simulink model "HumRob_V8"  (R2018a)
settings: Solver=FixedStepDiscrete  StartTime=0.0  StopTime=30  FixedStep=SampleTime  RelTol=1e-3  EnableMultiTasking=on
model workspace (MAT data in the model file):
  sampleTime = Simulink.Parameter
  sampleTime.DataType = 'auto'
  sampleTime.Dimensions = [0 0]
values from neighbouring files (symbols this model uses):
  PHI_t = deg2rad(15)    [init.m]
  scaling = 100    [init.m]
  T_la = 0.2*scaling    (= 20)    [init.m]
  T_st = 0.4*scaling    (= 40)    [init.m]
  T_sw = 1.1*scaling    (= 110)    [init.m]
  T_ta = 0.3*scaling    (= 30)    [init.m]
undefined symbols (not defined in the file or in its folder): DiscIntNeverNeededParam
libraries: raspberrypilib x3, embdlinuxlib x2, simulink x1, dspswit3 x1
settings Model: SimulationMode=external  ExtModeEnableFloating=off  Creator=t21st  LastModifiedBy=Kevin
settings SolverCC: PositivePriorityOrder=on  AutoInsertRateTranBlk=on  InsertRTBMode=Never (minimum delay)
settings DataIOCC: LimitDataPoints=on  MaxDataPoints=1000000
settings OptimizationCC: EnhancedBackFolding=on  PassReuseOutputArgsAs=Individual arguments  MaxStackSize=64  OptimizeBlockOrder=speed  DifferentSizesBufferReuse=on  OptimizationCustomize=off
settings DebuggingCC: ParameterTunabilityLossMsg=error
settings HardwareCC: ProdBitPerPointer=32  ProdBitPerSizeT=32  ProdBitPerPtrDiffT=32  ProdLargestAtomicInteger=Long  ProdLargestAtomicFloat=Double  ProdWordSize=32  ProdHWDeviceType=ARM Compatible->ARM Cortex
settings SFSimCC: MATLABDynamicMemAlloc=off
settings RTWCC: SystemTargetFile=ert.tlc  HardwareBoard=Raspberry Pi  TLCOptions="-aInlineSetEventsForThisBaseRateFcn=TLC_FALSE -aSuppressMultiTaskScheduler=TLC_FALSE  -aRateBasedStepFcn=0"  TemplateMakefile=ert_default_tmf  GenerateReport=on  Toolchain=GNU GCC Raspberry Pi  BuildConfiguration=Faster Runs  IncludeHyperlinkInReport=on  LaunchReport=on  GenerateTraceInfo=on  GenerateTraceReport=on  GenerateTraceReportSl=on  GenerateTraceReportSf=on  GenerateTraceReportEml=on
settings CodeAppCC: ForceParamTrailComments=on  IgnoreCustomStorageClasses=off  OperatorAnnotations=on  SimulinkDataObjDesc=on  SFDataObjDesc=on  InsertBlockDesc=on
settings ERTTargetCC: MatFileLogging=on  SupportVariableSizeSignals=on

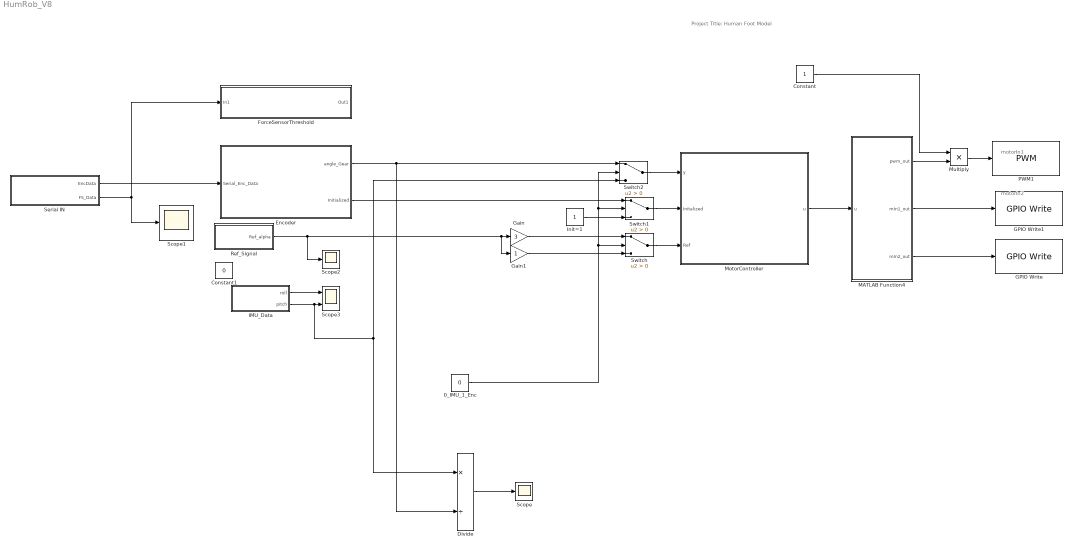
== system HumRob_V8 ==
  note: motorIn1
  note: motorIn2
  note: Project Title: Human Foot Model
  0_IMU_1_Enc : Constant  Value=0
  Constant : Constant
  Constant1 : Constant  Value=0
  Divide : Product  Inputs=*/
  Encoder : Subsystem
  ForceSensorThreshold : Subsystem
  GPIO Write : embdlinuxlib/GPIO Write  Description=asdf  board=Pi 3 Model B  gpio=24  direction=Output  blockPlatform=Raspberry Pi
      settings: SourceProductName=Simulink Support Package for Raspberry Pi Hardware  SourceProductBaseCode=RASPPI
  GPIO Write1 : embdlinuxlib/GPIO Write  board=Pi 3 Model B  gpio=23  direction=Output  blockPlatform=Raspberry Pi
      settings: SourceProductName=Simulink Support Package for Raspberry Pi Hardware  SourceProductBaseCode=RASPPI
  Gain : Gain  Gain=3
  Gain1 : Gain
  IMU_Data : Subsystem
  Init=1 : Constant
  MATLAB Function4 : MATLAB Function  TreatAsAtomicUnit=on
  MotorController : Subsystem
  Multiply : Product
  PWM1 : raspberrypilib/PWM  board=Pi 3 Model B  Pin_=18  Frequency=1000  blockPlatform=Raspberry Pi
      settings: SourceProductName=Simulink Support Package for Raspberry Pi Hardware  SourceProductBaseCode=RASPPI
  Ref_Signal : Subsystem
  Scope : Scope
  Scope1 : Scope
  Scope2 : Scope
  Scope3 : Scope  NumInputPorts=2
  Serial IN : Subsystem
  Switch : Switch  Criteria=u2 > Threshold
  Switch1 : Switch  Criteria=u2 > Threshold
  Switch2 : Switch  Criteria=u2 > Threshold
  wires:
  MATLAB Function4/2(mIn1_out) -> GPIO Write1/1
  MATLAB Function4/3(mIn2_out) -> GPIO Write/1
  MATLAB Function4/1(pwm_out) -> Multiply/2
  Multiply/1 -> PWM1/1
  Encoder/1("angle_Gear ") -> Switch2/1, Divide/2
  Encoder/2(Initialized) -> Switch1/1
  Gain/1 -> Switch/1
  MotorController/1(u) -> MATLAB Function4/1(u)
  Serial IN/2(FS_Data) -> ForceSensorThreshold/1(In1), Scope1/1
  Ref_Signal/1(Ref_alpha) -> Scope2/1, Gain1/1, Gain/1
  Serial IN/1("EncData ") -> Encoder/1(Serial_Enc_Data)
  IMU_Data/2(pitch) -> Divide/1, Switch2/3, Scope3/2
  IMU_Data/1(roll) -> Scope3/1
  Constant/1 -> Multiply/1
  Switch/1 -> MotorController/3(Ref)
  Gain1/1 -> Switch/3
  0_IMU_1_Enc/1 -> Switch2/2, Switch1/2, Switch/2
  Init=1/1 -> Switch1/3
  Switch2/1 -> MotorController/1(y)
  Switch1/1 -> MotorController/2(Initalized)
  Divide/1 -> Scope/1

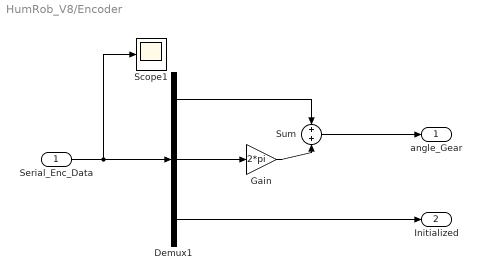
== system HumRob_V8/Encoder ==
  Serial_Enc_Data : Inport
  Demux1 : Demux  Outputs=3
  Gain : Gain  Gain=2*pi
  Scope1 : Scope
  Sum : Sum  Inputs=+|+
  "angle_Gear " : Outport
  Initialized : Outport  Port=2
  wires:
  Demux1/2 -> Gain/1
  Demux1/1 -> Sum/1
  Gain/1 -> Sum/2
  Sum/1 -> "angle_Gear "/1
  Demux1/3 -> Initialized/1
  Serial_Enc_Data/1 -> Scope1/1, Demux1/1

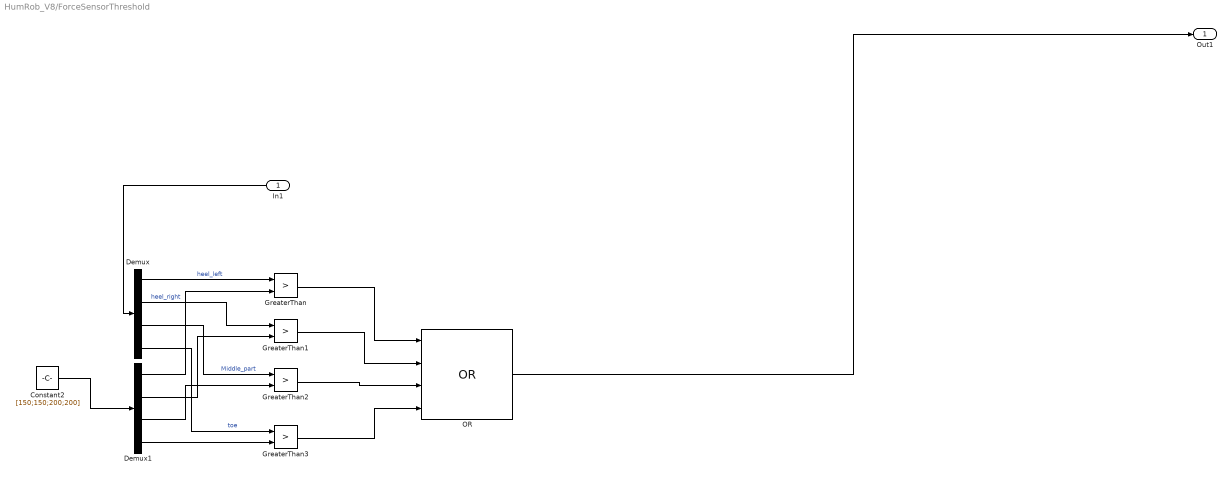
== system HumRob_V8/ForceSensorThreshold ==
  In1 : Inport
  Constant2 : Constant  Value=[150;150;200;200]
  Demux : Demux
  Demux1 : Demux
  GreaterThan{,1..3} (4 alike) : RelationalOperator  Operator=>  OutDataTypeStr=boolean  RndMeth=Simplest
  OR : Logic  Operator=OR  Inputs=4  IconShape=distinctive  AllPortsSameDT=off  OutDataTypeStr=boolean
  Out1 : Outport
  wires:
  Demux/3 -> GreaterThan2/1  "Middle_part"
  Demux1/2 -> GreaterThan1/2
  GreaterThan3/1 -> OR/4
  Demux/4 -> GreaterThan3/1  "toe"
  GreaterThan2/1 -> OR/3
  GreaterThan1/1 -> OR/2
  Demux/2 -> GreaterThan1/1  "heel_right"
  GreaterThan/1 -> OR/1
  Demux1/1 -> GreaterThan/2
  Demux/1 -> GreaterThan/1  "heel_left"
  Demux1/3 -> GreaterThan2/2
  Demux1/4 -> GreaterThan3/2
  OR/1 -> Out1/1
  Constant2/1 -> Demux1/1
  In1/1 -> Demux/1

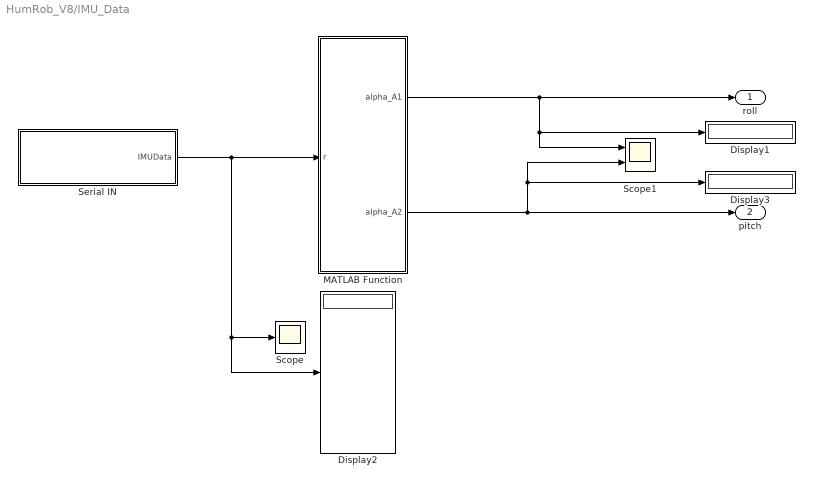
== system HumRob_V8/IMU_Data ==
  Display1 : Display
  Display2 : Display
  Display3 : Display
  MATLAB Function : MATLAB Function  TreatAsAtomicUnit=on
  Scope : Scope
  Scope1 : Scope  NumInputPorts=2
  Serial IN : Subsystem
  roll : Outport
  pitch : Outport  Port=2
  wires:
  Serial IN/1("IMUData ") -> Scope/1, Display2/1, MATLAB Function/1(r)
  MATLAB Function/1(alpha_A1) -> roll/1, Scope1/1, Display1/1
  MATLAB Function/2(alpha_A2) -> pitch/1, Scope1/2, Display3/1

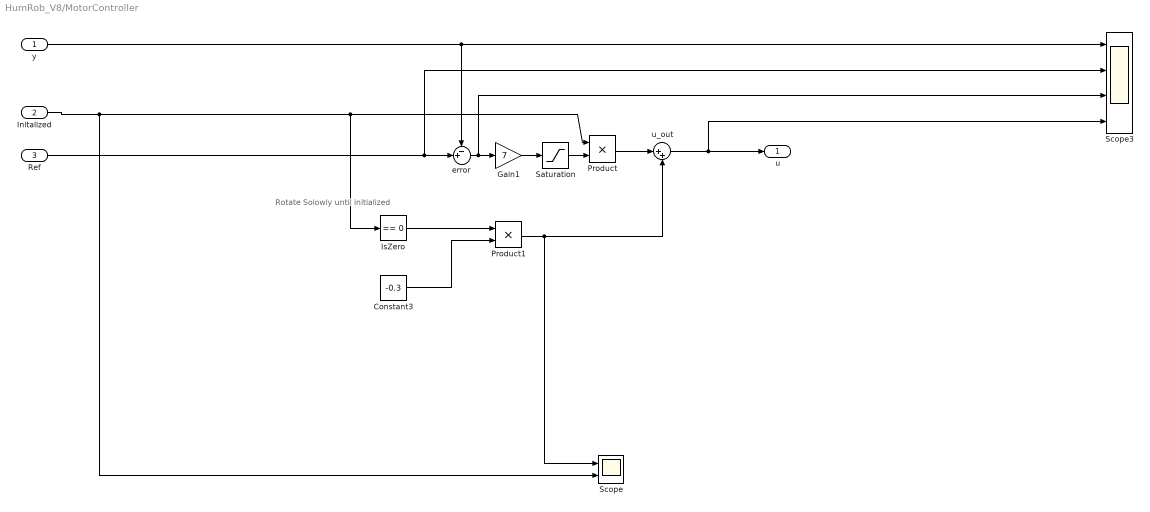
== system HumRob_V8/MotorController ==
  note: Rotate Solowly until initialized
  y : Inport
  Initalized : Inport  Port=2
  Ref : Inport  Port=3
  Constant3 : Constant  Value=-0.3
  Gain1 : Gain  Gain=7
  IsZero : simulink/Logic and Bit Operations/Compare To Zero  relop===  OutDataTypeStr=boolean
  Product : Product
  Product1 : Product
  Saturation : Saturate  UpperLimit=1  LowerLimit=-1
  Scope : Scope  NumInputPorts=2
  Scope3 : Scope  NumInputPorts=4
  error : Sum  Inputs=-+|
  u_out : Sum  Inputs=|++
  u : Outport
  wires:
  Gain1/1 -> Saturation/1
  Product/1 -> u_out/1
  error/1 -> Scope3/3, Gain1/1
  Saturation/1 -> Product/2
  y/1 -> error/1, Scope3/1
  Product1/1 -> Scope/1, u_out/2
  u_out/1 -> Scope3/4, u/1
  Constant3/1 -> Product1/2
  IsZero/1 -> Product1/1
  Ref/1 -> Scope3/2, error/2
  Initalized/1 -> Scope/2, IsZero/1, Product/1

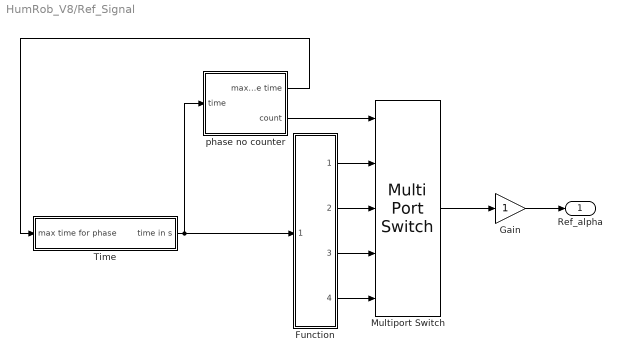
== system HumRob_V8/Ref_Signal ==
  Function : Subsystem
  Gain : Gain
  Multiport Switch : MultiPortSwitch  Inputs=4
  "Time " : Subsystem
  phase no counter : Subsystem
  Ref_alpha : Outport
  wires:
  "Time "/1(time in s) -> Function/1(time), phase no counter/1(time)
  Function/2(take off) -> Multiport Switch/3
  Function/1(stand) -> Multiport Switch/2
  phase no counter/2(count) -> Multiport Switch/1
  Function/4(land) -> Multiport Switch/5
  Function/3(swing) -> Multiport Switch/4
  phase no counter/1(max phase time) -> "Time "/1(max time for phase)
  Multiport Switch/1 -> Gain/1
  Gain/1 -> Ref_alpha/1

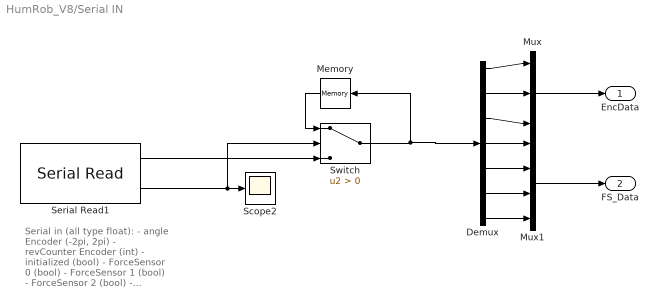
== system HumRob_V8/Serial IN ==
  note: Serial in (all type float):
      | - angle Encoder (-2pi, 2pi)
      | - revCounter Encoder (int)
      | - initialized (bool)
      |
      | - ForceSensor 0 (bool)
      | - ForceSensor 1 (bool)
      | - ForceSensor 2 (bool)
      | - ForceSensor 3 (bool)
  Demux : Demux  Outputs=7
  Memory : Memory
  Mux : Mux  Inputs=3
  Mux1 : Mux
  Scope2 : Scope
  Serial Read1 : raspberrypilib/Serial Read  board=Pi 3 Model B  SCIModule_=/dev/ttyUSB0  Baudrate_=230400  Parity=None  StopBits_=1  HardwareFlowControl=None  ByteOrder=LittleEndian  DataLength=7  DataType=single  OutputStatus=on  SampleTime=-1  blockPlatform=RaspberryPi
      settings: SourceProductName=Simulink Support Package for Raspberry Pi Hardware  SourceProductBaseCode=RASPPI
  Switch : Switch  Criteria=u2 > Threshold
  "EncData " : Outport
  FS_Data : Outport  Port=2
  wires:
  Serial Read1/2 -> Switch/2, Scope2/1
  Memory/1 -> Switch/1
  Serial Read1/1 -> Switch/3
  Switch/1 -> Demux/1, Memory/1
  Demux/1 -> Mux/1
  Demux/2 -> Mux/2
  Demux/3 -> Mux/3
  Demux/4 -> Mux1/1
  Demux/5 -> Mux1/2
  Demux/6 -> Mux1/3
  Demux/7 -> Mux1/4
  Mux/1 -> "EncData "/1
  Mux1/1 -> FS_Data/1

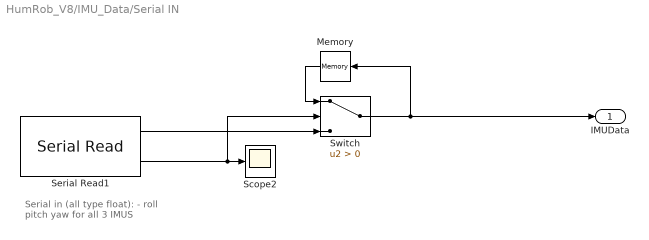
== system HumRob_V8/IMU_Data/Serial IN ==
  note: Serial in (all type float):
      | - roll pitch yaw for all 3 IMUS
  Memory : Memory
  Scope2 : Scope
  Serial Read1 : raspberrypilib/Serial Read  board=Pi 3 Model B  SCIModule_=/dev/ttyACM0  Baudrate_=230400  Parity=None  StopBits_=1  HardwareFlowControl=None  ByteOrder=LittleEndian  DataLength=9  DataType=single  OutputStatus=on  SampleTime=-1  blockPlatform=RaspberryPi
      settings: SourceProductName=Simulink Support Package for Raspberry Pi Hardware  SourceProductBaseCode=RASPPI
  Switch : Switch  Criteria=u2 > Threshold
  "IMUData " : Outport
  wires:
  Serial Read1/2 -> Switch/2, Scope2/1
  Memory/1 -> Switch/1
  Serial Read1/1 -> Switch/3
  Switch/1 -> Memory/1, "IMUData "/1

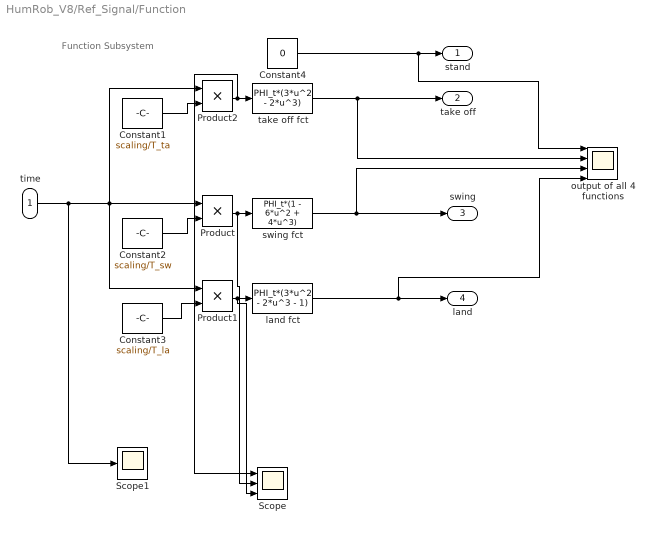
== system HumRob_V8/Ref_Signal/Function ==
  note: Function Subsystem
  time : Inport
  Constant1 : Constant  Value=scaling/T_ta
  Constant2 : Constant  Value=scaling/T_sw
  Constant3 : Constant  Value=scaling/T_la
  Constant4 : Constant  Value=0
  Product : Product
  Product1 : Product
  Product2 : Product
  Scope : Scope  NumInputPorts=3
  Scope1 : Scope
  land fct : Fcn  Expr=PHI_t*(3*u^2 - 2*u^3 - 1)
  output of all 4 functions : Scope  NumInputPorts=4
  swing fct : Fcn  Expr=PHI_t*(1 - 6*u^2 + 4*u^3)
  take off fct : Fcn  Expr=PHI_t*(3*u^2 - 2*u^3)
  stand : Outport
  take off : Outport  Port=2
  swing : Outport  Port=3
  land : Outport  Port=4
  wires:
  time/1 -> Scope1/1, Product/1, Product2/1, Product1/1
  Constant4/1 -> output of all 4 functions/1, stand/1
  Product/1 -> Scope/2, swing fct/1
  Constant2/1 -> Product/2
  land fct/1 -> output of all 4 functions/4, land/1
  Constant3/1 -> Product1/2
  Product1/1 -> Scope/3, land fct/1
  swing fct/1 -> output of all 4 functions/3, swing/1
  take off fct/1 -> output of all 4 functions/2, take off/1
  Product2/1 -> Scope/1, take off fct/1
  Constant1/1 -> Product2/2

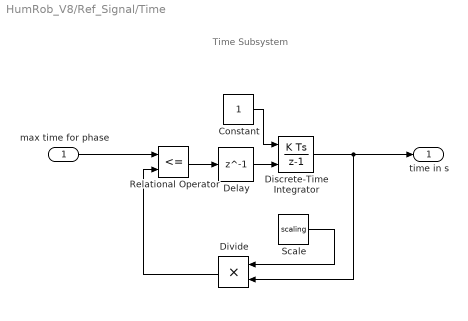
== system HumRob_V8/Ref_Signal/Time  ==
  note: Time Subsystem
  max time for phase : Inport
  Constant : Constant
  Delay : Delay  DelayLength=1
  Discrete-Time Integrator : DiscreteIntegrator  ExternalReset=rising  SampleTime=-1  ICPrevOutput=DiscIntNeverNeededParam  ICPrevScaledInput=DiscIntNeverNeededParam
  Divide : Product  Inputs=**
  Relational Operator : RelationalOperator  Operator=<=  OutDataTypeStr=boolean  RndMeth=Nearest
  Scale : Constant  Value=scaling
  time in s : Outport
  wires:
  Discrete-Time Integrator/1 -> time in s/1, Divide/2
  Relational Operator/1 -> Delay/1
  max time for phase/1 -> Relational Operator/1
  Delay/1 -> Discrete-Time Integrator/2
  Constant/1 -> Discrete-Time Integrator/1
  Scale/1 -> Divide/1
  Divide/1 -> Relational Operator/2

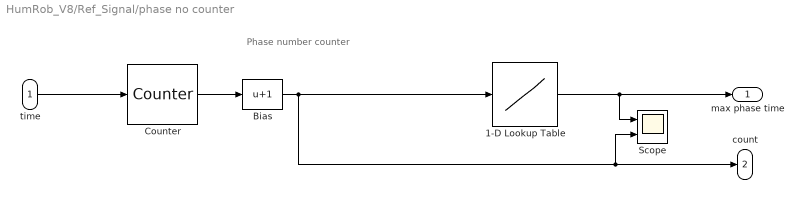
== system HumRob_V8/Ref_Signal/phase no counter ==
  note: Phase number counter
  time : Inport
  1-D Lookup Table : Lookup_n-D  NumberOfTableDimensions=1  BreakpointsForDimension1=[1,2,3,4]  BreakpointsForDimension1FirstPoint=10  BreakpointsForDimension2FirstPoint=10  BreakpointsForDimension1Spacing=12  BreakpointsForDimension2Spacing=12  IndexSearchMethod=Evenly spaced points  Table=[T_st,T_ta,T_sw,T_la]  InterpMethod=Flat  DiagnosticForOutOfRangeInput=Error  InternalRulePriority=Speed  RndMeth=Simplest  InputSameDT=on
  Bias : Bias  Bias=1
  Counter : dspswit3/Counter  Direction=Up  CountEvent=Falling edge  CounterSize=User defined  MaxCount=3  InitialCount=0  Output=Count  HitValue=32  ResetInput=off  SamplesPerFrame=1  Ts=1  CntDtype=int8  HitDtype=Logical
  Scope : Scope  NumInputPorts=2
  max phase time : Outport
  count : Outport  Port=2
  wires:
  Counter/1 -> Bias/1
  Bias/1 -> Scope/2, count/1, 1-D Lookup Table/1
  time/1 -> Counter/1
  1-D Lookup Table/1 -> Scope/1, max phase time/1

== matlab function HumRob_V8/IMU_Data/MATLAB Function ==
  data: r input; alpha_A1 output; alpha_A2 output
function [alpha_A1, alpha_A2] = fcn(r)

rx1 = r(1);
rx2 = r(4);
rx3 = r(7);

ry1 = r(2);
ry2 = r(5);
ry3 = r(8);

rz1 = r(3);
rz2 = r(6);
rz3 = r(9);

Rxa1 = Rx(rx1);
Ryb1 = Ry(ry1);
Rzc1 = Rz(rz1);
R_G_IMU_1 = Rzc1*Ryb1*Rxa1;
R_G_IMU_1 = R_G_IMU_1(1:3,1:3);
R_IMU1_G = R_G_IMU_1';
%z_G_IMU1 = R_IMU1_G(1:3,3); %z Axis of G System in IMU System


Rxa2 = Rx(rx2);
Ryb2 = Ry(ry2);
Rzc2 = Rz(rz2);
R_G_IMU_2 = Rzc2*Ryb2*Rxa2;
R_G_IMU_2 = R_G_IMU_2(1:3,1:3);
R_IMU2_G = R_G_IMU_2';
%z_G_IMU2 = R_IMU2_G(1:3,3); %z Axis of G System in IMU System


Rxa3 = Rx(rx3);
Ryb3 = Ry(ry3);
Rzc3 = Rz(rz3);
R_G_IMU_3 = Rzc3*Ryb3*Rxa3;
R_G_IMU_3 = R_G_IMU_3(1:3,1:3);
R_IMU3_G = R_G_IMU_3';
%z_G_IMU3 = R_IMU3_G(1:3,3); %z Axis of G System in IMU System

%alpha_IMU = acos((dot(z_G_IMU2,z_G_IMU3))/(norm(z_G_IMU2)*norm(z_G_IMU2)))*180/pi;

R_IMU1_A11 = [0 0 -1; 1 0 0; 0 -1 0];
R_IMU2_A12 = [0 0 -1; 1 0 0; 0 -1 0];

R_IMU2_A22 = [-1 0 0; 0 0 1; 0 1 0 ];
R_IMU3_A23 = [-1 0 0; 0 0 -1; 0 -1 0];



%R_A22_A23 = R_IMU2_A22' * R_G_IMU_2' * R_G_IMU_3 *R_IMU3_A23
R_A11_G = R_IMU1_A11' * R_IMU1_G;
R_A12_G = R_IMU2_A12' * R_IMU2_G;
R_A22_G = R_IMU2_A22' * R_IMU2_G;
R_A23_G = R_IMU3_A23' * R_IMU3_G;

z_G_A11 = R_A11_G(1:3,3);
z_G_A12 = R_A12_G(1:3,3);
z_G_A22 = R_A22_G(1:3,3);
z_G_A23 = R_A23_G(1:3,3);


alpha_A1 = acos((dot(z_G_A11,z_G_A12))/(norm(z_G_A11)*norm(z_G_A12)));
alpha_A2 = acos((dot(z_G_A22,z_G_A23))/(norm(z_G_A22)*norm(z_G_A23)));

cr12 = cross(z_G_A11,z_G_A12);
cr23 = cross(z_G_A22,z_G_A23);
s1 = sign(cr12(1));
s2 = sign(cr23(1));

alpha_A1 = s1 * alpha_A1;
alpha_A2 = s2 * alpha_A2;

end

== matlab function HumRob_V8/MATLAB Function4 ==
  data: u input; pwm_out output; mIn1_out output; mIn2_out output
function [pwm_out,mIn1_out,mIn2_out] = motorControl(u)
%   initial signals
pwm_out=0
% limits for pwm 0.3 to 1
PWM_LIMIT = 0.3;
%         Turn left
if(-1 <= u && u <= -PWM_LIMIT)
%     display('Turn Left: ')
    pwm_out = abs(u)
    mIn1_out = 1
    mIn2_out = 0
    %     motor stop
elseif(-PWM_LIMIT < u && u < PWM_LIMIT)
%     display('Motor Stop: ')
    pwm_out = 0
    mIn1_out = 1
    mIn2_out = 1
    %     motor turn right
elseif (PWM_LIMIT <= u && u <= 1)
%     display('Motor turn right: ')
    pwm_out = abs(u)
    mIn1_out = 0
    mIn2_out = 1
else
    %     motor stop
%     display('Motor EMERGENCY')
    pwm_out = 0
    mIn1_out = 1
    mIn2_out = 1
end
